simulink model "week_4"  (R2024a)
settings: Solver=VariableStepAuto  StartTime=0.0  StopTime=10  RelTol=1e-3
values from neighbouring files (symbols this model uses):
  J = 0.02    [ControlSystemFinal_ChoiChiHyuk.m]
  K = acker(A,B,desired_poles)    [ControlSystemFinal_ChoiChiHyuk.m]
  K_syme = acker(A,B,desired_poles_syme)    [ControlSystemFinal_ChoiChiHyuk.m]
  Kb = 0.015    [ControlSystemFinal_ChoiChiHyuk.m]
  Kf = 0.2    [ControlSystemFinal_ChoiChiHyuk.m]
  Km = 0.015    [ControlSystemFinal_ChoiChiHyuk.m]
  L = 0.5    [ControlSystemFinal_ChoiChiHyuk.m]
  Nb = Nu+K*Nx    [ControlSystemFinal_ChoiChiHyuk.m]
  Nb_syme = Nu + K_syme*Nx    [ControlSystemFinal_ChoiChiHyuk.m]
  R = 2.0    (= 2)    [ControlSystemFinal_ChoiChiHyuk.m]
settings Model: Creator=CHI  LastModifiedBy=CHI

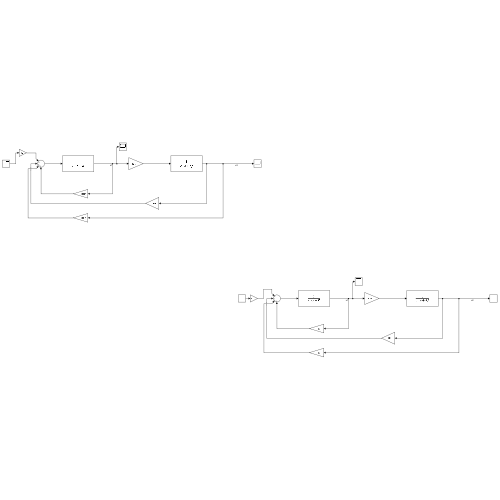
[thumbnail: Simulink's stored preview of the top-level diagram]
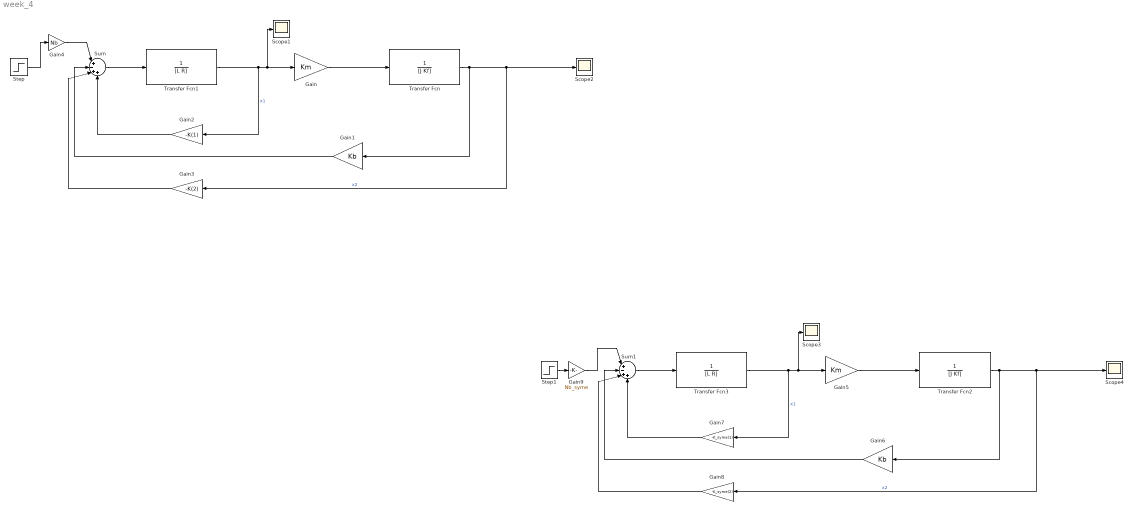
== system week_4 ==
  Gain : Gain  Gain=Km
  Gain1 : Gain  Gain=Kb
  Gain2 : Gain  Gain=-K(1)
  Gain3 : Gain  Gain=-K(2)
  Gain4 : Gain  Gain=Nb
  Gain5 : Gain  Gain=Km
  Gain6 : Gain  Gain=Kb
  Gain7 : Gain  Gain=-K_syme(1)
  Gain8 : Gain  Gain=-K_syme(2)
  Gain9 : Gain  Gain=Nb_syme
  Scope{1..4} (4 alike) : Scope
  Step : Step  SampleTime=0
  Step1 : Step  SampleTime=0
  Sum : Sum  Inputs=|+-++
  Sum1 : Sum  Inputs=|+-++
  Transfer Fcn : TransferFcn  Denominator=[J Kf]
  Transfer Fcn1 : TransferFcn  Denominator=[L R]
  Transfer Fcn2 : TransferFcn  Denominator=[J Kf]
  Transfer Fcn3 : TransferFcn  Denominator=[L R]
  wires:
  Transfer Fcn/1 -> Gain3/1, Scope2/1, Gain1/1  "x2"
  Gain/1 -> Transfer Fcn/1
  Gain1/1 -> Sum/2
  Sum/1 -> Transfer Fcn1/1
  Transfer Fcn1/1 -> Gain2/1, Scope1/1, Gain/1  "x1"
  Gain2/1 -> Sum/4
  Gain3/1 -> Sum/3
  Step/1 -> Gain4/1
  Gain4/1 -> Sum/1
  Gain9/1 -> Sum1/1
  Sum1/1 -> Transfer Fcn3/1
  Transfer Fcn3/1 -> Gain7/1, Scope3/1, Gain5/1  "x1"
  Step1/1 -> Gain9/1
  Gain8/1 -> Sum1/3
  Gain7/1 -> Sum1/4
  Gain5/1 -> Transfer Fcn2/1
  Transfer Fcn2/1 -> Gain8/1, Scope4/1, Gain6/1  "x2"
  Gain6/1 -> Sum1/2
